simulink model "dc_motor_SL"  (R2024b)
settings: Solver=VariableStepAuto  StartTime=0.0  StopTime=10.0  RelTol=1e-3
PreLoadFcn:
  | load properties.mat
values from neighbouring files (symbols this model uses):
  K = 0.1    [properties.mat]
  L = 0.5    [properties.mat]
  R = 1    [properties.mat]
  V = 12    [properties.mat]
settings Model: Creator=garellan  LastModifiedBy=garellan

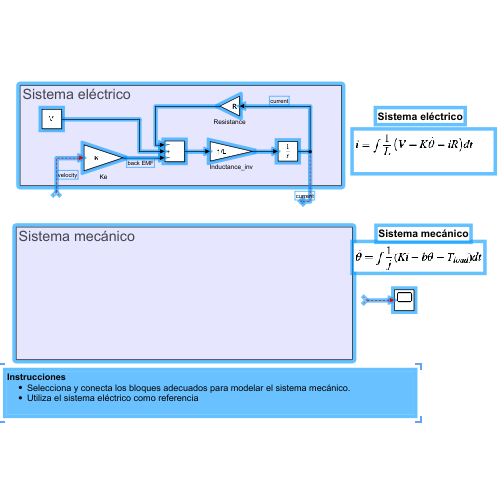
[thumbnail: Simulink's stored preview of the top-level diagram]
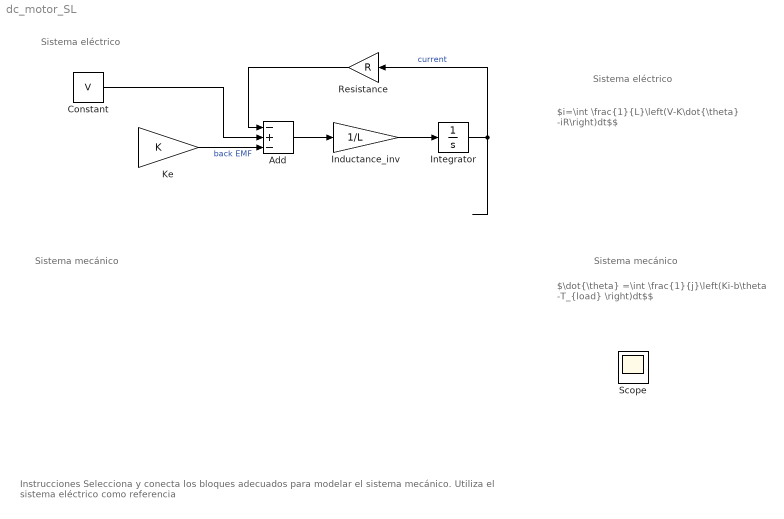
== system dc_motor_SL ==
  note: Sistema mecánico
  note: Sistema eléctrico
  note: $i=\int \frac{1}{L}\left(V-K\dot{\theta} -iR\right)dt$$
  note: Sistema eléctrico
  note: Sistema mecánico
  note: $\dot{\theta} =\int \frac{1}{j}\left(Ki-b\theta -T_{load} \right)dt$$
  note: Instrucciones
      | Selecciona y conecta los bloques adecuados para modelar el sistema mecánico.
      | Utiliza el sistema eléctrico como referencia
  Add : Sum  Inputs=-+-
  Constant : Constant  Value=V
  Inductance_inv : Gain  Gain=1/L
  Integrator : Integrator
  Ke : Gain  Gain=K
  Resistance : Gain  Gain=R
  Scope : Scope
  wires:
  ? -> Scope/1
  Constant/1 -> Add/2
  Ke/1 -> Add/3  "back EMF"
  Integrator/1 -> Resistance/1  "current"
  Inductance_inv/1 -> Integrator/1
  ? -> Ke/1  "velocity"
  Resistance/1 -> Add/1
  Add/1 -> Inductance_inv/1
